simulink model "chapter4"  (R2018b)
settings: Solver=VariableStepAuto  StartTime=0.0  StopTime=10  RelTol=1e-3
undefined symbols (not defined in the file): sigbuilder_block
libraries: simulink x2
settings Model: Creator=nharada  LastModifiedBy=nharada

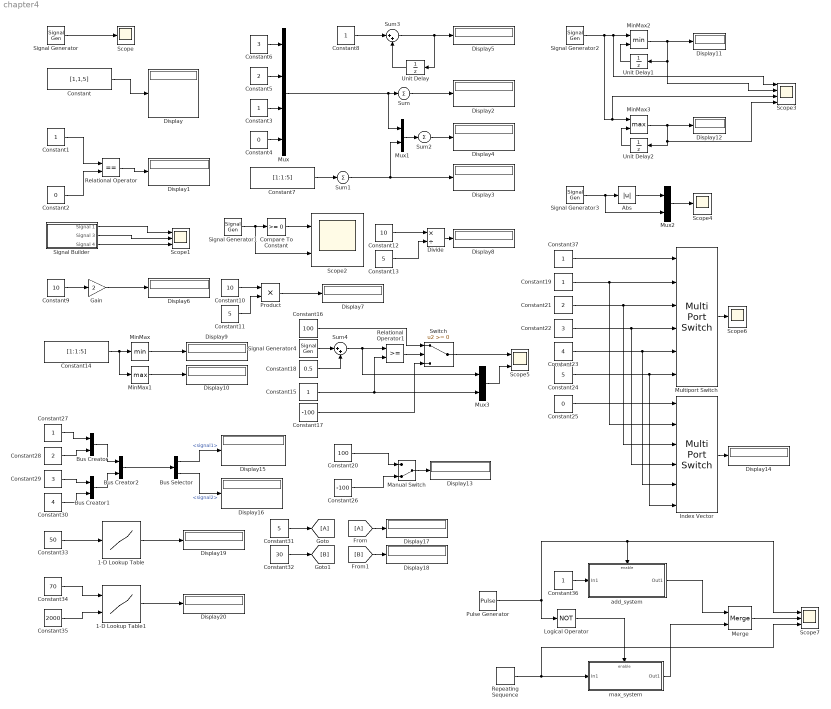
== system chapter4 ==
  1-D Lookup Table : Lookup_n-D  NumberOfTableDimensions=1  BreakpointsForDimension1=[0 50 100]  Table=[0 3500 7000]  InternalRulePriority=Speed  RndMeth=Simplest  InputSameDT=on
  1-D Lookup Table1 : Lookup_n-D  BreakpointsForDimension1=[0,10,50,100]  BreakpointsForDimension2=[0,3500,7000]  Table=reshape([0,0,0,0,50,75,100,200,100,150,200,400],4,3)  InternalRulePriority=Speed  RndMeth=Simplest  InputSameDT=on
  Abs : Abs
  Bus Creator : BusCreator  Inputs=2
  Bus Creator1 : BusCreator  Inputs=2
  Bus Creator2 : BusCreator  Inputs=2
  Bus Selector : BusSelector  OutputSignals=signal1,signal2
  Compare To Constant : simulink/Logic and Bit Operations/Compare To Constant  relop=>=  const=0  OutDataTypeStr=boolean
  Constant : Constant  Value=[1,1,5]
  Constant{1,3,15,19,27,37} (6 alike) : Constant
  Constant10 : Constant  Value=10  SampleTime=1
  Constant11 : Constant  Value=5  SampleTime=1
  Constant12 : Constant  Value=10  SampleTime=1
  Constant13 : Constant  Value=5  SampleTime=1
  Constant14 : Constant  Value=[1:1:5]
  Constant16 : Constant  Value=100
  Constant17 : Constant  Value=-100
  Constant18 : Constant  Value=0.5  SampleTime=1
  Constant2 : Constant  Value=0
  Constant20 : Constant  Value=100
  Constant21 : Constant  Value=2
  Constant22 : Constant  Value=3
  Constant23 : Constant  Value=4
  Constant24 : Constant  Value=5
  Constant25 : Constant  Value=0
  Constant26 : Constant  Value=-100
  Constant28 : Constant  Value=2
  Constant29 : Constant  Value=3
  Constant30 : Constant  Value=4
  Constant31 : Constant  Value=5
  Constant32 : Constant  Value=30
  Constant33 : Constant  Value=50
  Constant34 : Constant  Value=70
  Constant35 : Constant  Value=2000
  Constant36 : Constant  SampleTime=0.001
  Constant4 : Constant  Value=0
  Constant5 : Constant  Value=2
  Constant6 : Constant  Value=3
  Constant7 : Constant  Value=[1:1:5]
  Constant8 : Constant  SampleTime=1
  Constant9 : Constant  Value=10  SampleTime=1
  Display{,1..20} (21 alike) : Display
  Divide : Product  Inputs=*/
  Gain : Gain  Gain=2
  Index Vector : MultiPortSwitch  DataPortOrder=Zero-based contiguous  Inputs=5  zeroidx=on
  Logical Operator : Logic  Operator=NOT  Inputs=1  AllPortsSameDT=off  OutDataTypeStr=boolean
  Manual Switch : ManualSwitch  CurrentSetting=0
  Merge : Merge
  MinMax : MinMax
  MinMax1 : MinMax  Function=max
  MinMax2 : MinMax  Inputs=2
  MinMax3 : MinMax  Function=max  Inputs=2
  Multiport Switch : MultiPortSwitch  Inputs=5
  Mux : Mux
  Mux1 : Mux  Inputs=2
  Mux2 : Mux  Inputs=2
  Mux3 : Mux  Inputs=2
  Product : Product
  Pulse Generator : DiscretePulseGenerator  PulseType=Time based  PulseWidth=50
  Relational Operator : RelationalOperator  Operator===  OutDataTypeStr=boolean  RndMeth=Simplest
  Relational Operator1 : RelationalOperator  OutDataTypeStr=fixdt(1,16)  RndMeth=Simplest
  Repeating Sequence : simulink/Sources/Repeating Sequence  rep_seq_t=[0 2]  rep_seq_y=[0 5]
  Scope : Scope
  Scope1 : Scope  NumInputPorts=3
  Scope2 : Scope  NumInputPorts=2
  Scope3 : Scope  NumInputPorts=4
  Scope4 : Scope
  Scope5 : Scope  NumInputPorts=2
  Scope6 : Scope
  Scope7 : Scope  NumInputPorts=3
  Signal Generator : SignalGenerator  WaveForm=square  Frequency=100  Units=rad/sec
  Signal Generator1 : SignalGenerator  WaveForm=square  Frequency=10  Units=rad/sec
  Signal Generator2 : SignalGenerator  Frequency=0.1
  Signal Generator3 : SignalGenerator  Frequency=0.1
  Signal Generator4 : SignalGenerator  WaveForm=square  Amplitude=0.5  Frequency=0.1
  Signal Builder : Subsystem  Tag=STV Subsys  LoadFcn=sigbuilder_block('load');  StartFcn=sigbuilder_block('start');  StopFcn=sigbuilder_block('stop');  ClipboardFcn=sigbuilder_block('clipboard');  mask(Sigbuilder block){tuvar=[0:10]}
      mask help: Simulink:masks:SigbuilderBlock_MD
      mask init:
      | if ~strcmp(get_param(bdroot(gcbh),'SimulationStatus'),'stopped') tuvar = sigbuilder_block('maskInit'); end
      settings: CopyFcn=sigbuilder_block('copy');  DeleteFcn=sigbuilder_block('delete');  ModelCloseFcn=sigbuilder_block('modelClose');  PreSaveFcn=sigbuilder_block('preSave');  PauseFcn=sigbuilder_block('pause');  ContinueFcn=sigbuilder_block('continue');  NameChangeFcn=sigbuilder_block('namechange');  OpenFcn=sigbuilder_block('open',[437.6 199.2 550.4 400 ]);  CloseFcn=sigbuilder_block('close');
      mask Display: plot(0, 0, 100, 100,[2, 2, 32, 32, 2], [68, 8, 8, 68, 68],[32, 2], [38, 38], [32, 19, 2],[53, 60, 44], [32, 17, 17, 2],[16, 16, 31, 31]);txt = getActiveGroup(gcbh);text(2, 100, txt,'verticalAlignment', 'top');
  Sum : Sum  Inputs=+
  Sum1 : Sum  Inputs=+
  Sum2 : Sum  Inputs=+
  Sum3 : Sum  Inputs=|++
  Sum4 : Sum  Inputs=|++
  Switch : Switch
  Unit Delay : UnitDelay  SampleTime=-1
  Unit Delay1 : UnitDelay  SampleTime=-1
  Unit Delay2 : UnitDelay  SampleTime=-1
  add_system : Subsystem
  max_system : Subsystem
  wires:
  Constant/1 -> Display/1
  Signal Generator/1 -> Scope/1
  Signal Builder/1(Signal 1) -> Scope1/1
  Signal Builder/2(Signal 3) -> Scope1/2
  Signal Builder/3(Signal 4) -> Scope1/3
  Constant1/1 -> Relational Operator/1
  Constant2/1 -> Relational Operator/2
  Relational Operator/1 -> Display1/1
  Compare To Constant/1 -> Scope2/1
  Signal Generator1/1 -> Scope2/2, Compare To Constant/1
  Sum/1 -> Display2/1
  Mux/1 -> Mux1/1, Sum/1
  Constant3/1 -> Mux/3
  Constant4/1 -> Mux/4
  Constant6/1 -> Mux/1
  Constant5/1 -> Mux/2
  Sum1/1 -> Mux1/2, Display3/1
  Constant7/1 -> Sum1/1
  Mux1/1 -> Sum2/1
  Sum2/1 -> Display4/1
  Sum3/1 -> Unit Delay/1, Display5/1
  Constant8/1 -> Sum3/1
  Unit Delay/1 -> Sum3/2
  Constant9/1 -> Gain/1
  Gain/1 -> Display6/1
  Product/1 -> Display7/1
  Constant10/1 -> Product/1
  Constant11/1 -> Product/2
  Divide/1 -> Display8/1
  Constant12/1 -> Divide/1
  Constant13/1 -> Divide/2
  Constant14/1 -> MinMax1/1, MinMax/1
  MinMax/1 -> Display9/1
  MinMax1/1 -> Display10/1
  MinMax2/1 -> Scope3/2, Unit Delay1/1, Display11/1
  Unit Delay1/1 -> MinMax2/2
  Unit Delay2/1 -> MinMax3/2
  MinMax3/1 -> Unit Delay2/1, Scope3/4, Display12/1
  Signal Generator2/1 -> Scope3/3, MinMax3/1, Scope3/1, MinMax2/1
  Abs/1 -> Mux2/1
  Signal Generator3/1 -> Mux2/2, Abs/1
  Mux2/1 -> Scope4/1
  Switch/1 -> Scope5/1
  Relational Operator1/1 -> Switch/2
  Constant15/1 -> Relational Operator1/2, Mux3/2
  Constant16/1 -> Switch/1
  Constant17/1 -> Switch/3
  Mux3/1 -> Scope5/2
  Constant18/1 -> Sum4/2
  Signal Generator4/1 -> Sum4/1
  Sum4/1 -> Relational Operator1/1, Mux3/1
  Constant37/1 -> Multiport Switch/1
  Constant19/1 -> Multiport Switch/2, Index Vector/2
  Constant21/1 -> Multiport Switch/3, Index Vector/3
  Constant22/1 -> Multiport Switch/4, Index Vector/4
  Constant23/1 -> Index Vector/5, Multiport Switch/5
  Constant24/1 -> Index Vector/6, Multiport Switch/6
  Multiport Switch/1 -> Scope6/1
  Index Vector/1 -> Display14/1
  Constant25/1 -> Index Vector/1
  Constant20/1 -> Manual Switch/1
  Constant26/1 -> Manual Switch/2
  Manual Switch/1 -> Display13/1
  Constant27/1 -> Bus Creator/1
  Constant28/1 -> Bus Creator/2
  Constant29/1 -> Bus Creator1/1
  Constant30/1 -> Bus Creator1/2
  Bus Creator2/1 -> Bus Selector/1
  Bus Creator/1 -> Bus Creator2/1
  Bus Creator1/1 -> Bus Creator2/2
  Bus Selector/1 -> Display15/1  "<signal1>"
  Bus Selector/2 -> Display16/1  "<signal2>"
  Constant31/1 -> [A]
  [A] -> Display17/1
  [B] -> Display18/1
  Constant32/1 -> [B]
  Constant33/1 -> 1-D Lookup Table/1
  1-D Lookup Table/1 -> Display19/1
  1-D Lookup Table1/1 -> Display20/1
  Constant34/1 -> 1-D Lookup Table1/1
  Constant35/1 -> 1-D Lookup Table1/2
  Pulse Generator/1 -> Logical Operator/1, Scope7/1, add_system/Enable
  Repeating Sequence/1 -> Scope7/3, max_system/1(In1)
  Merge/1 -> Scope7/2
  Constant36/1 -> add_system/1(In1)
  add_system/1(Out1) -> Merge/1
  max_system/1(Out1) -> Merge/2
  Logical Operator/1 -> max_system/Enable

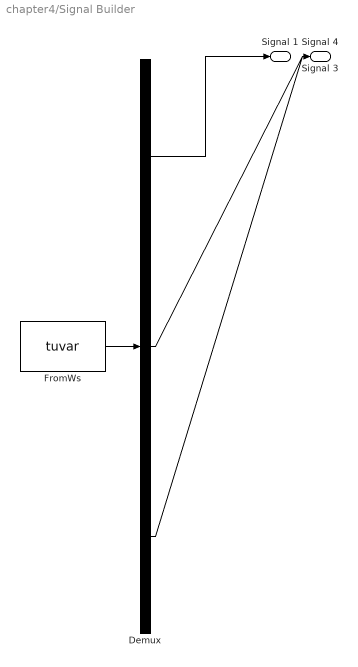
== system chapter4/Signal Builder ==
  Demux : Demux  Tag=STV Demux  Outputs=3
  FromWs : FromWorkspace  Tag=STV FromWs  VariableName=tuvar  SampleTime=0
      SigBuilderData=|
      | common.afterFinalStr = 'Extrapolate'
      | common.sampleTime = 0
      | dataSet.timeRange = [0 10]
      | dataSet.name = 'Group 4'
      | sbobj.Groups.Name = 'Group 4'
      | sbobj.Groups.Signals(1).Name = 'Signal 1'
      | sbobj.Groups.Signals(1).XData = [0 4 4 6 6 10]
      | sbobj.Groups.Signals(1).YData = [0 0 1 1 0 0]
      | sbobj.Groups.Signals(2).Name = 'Signal 3'
      | sbobj.Groups.Signals(2).XData = [0 0.0204081632653 0.0408163265306 0.0612244897959 0.0816326530612 0.102040816327 0.122448979592 0.142857142857 0.163265306122 0.183673469388 0.204081632653 0.224489795918 ... (491 elements, 1x491)]
      | sbobj.Groups.Signals(2).YData = [1 1.12787716168 1.25365458391 1.37526700488 1.490717552 1.59811053049 1.6956825506 1.78183148247 1.85514276301 1.91441262302 1.95866785304 1.98718178341 ... (491 elements, 1x491)]
      | sbobj.Groups.Signals(3).Name = 'Signal 4'
      | sbobj.Groups.Signals(3).XData = [0 5 5 10]
      | sbobj.Groups.Signals(3).YData = [0 0 1 1]
  Signal 1 : Outport  Tag=STV Outport
  Signal 3 : Outport  Tag=STV Outport  Port=2
  Signal 4 : Outport  Tag=STV Outport  Port=3
  wires:
  Demux/1 -> Signal 1/1
  FromWs/1 -> Demux/1
  Demux/2 -> Signal 3/1
  Demux/3 -> Signal 4/1

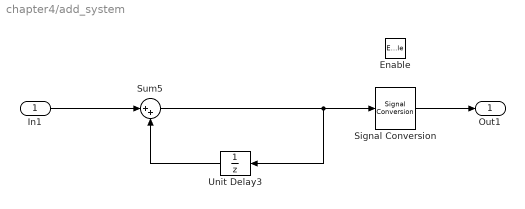
== system chapter4/add_system ==
  In1 : Inport
  Enable : EnablePort  StatesWhenEnabling=reset
  Signal Conversion : SignalConversion  OverrideOpt=off
  Sum5 : Sum  Inputs=|++
  Unit Delay3 : UnitDelay  SampleTime=-1
  Out1 : Outport
  wires:
  Unit Delay3/1 -> Sum5/2
  Sum5/1 -> Unit Delay3/1, Signal Conversion/1
  In1/1 -> Sum5/1
  Signal Conversion/1 -> Out1/1

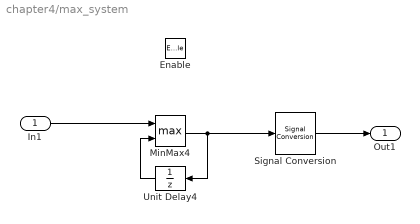
== system chapter4/max_system ==
  In1 : Inport
  Enable : EnablePort  StatesWhenEnabling=reset
  MinMax4 : MinMax  Function=max  Inputs=2
  Signal Conversion : SignalConversion  OverrideOpt=off
  Unit Delay4 : UnitDelay  SampleTime=-1
  Out1 : Outport
  wires:
  Unit Delay4/1 -> MinMax4/2
  In1/1 -> MinMax4/1
  MinMax4/1 -> Signal Conversion/1, Unit Delay4/1
  Signal Conversion/1 -> Out1/1
